simulink model "Slip_compensation_model"  (R2019b)
settings: Solver=VariableStepAuto  StartTime=0.0  StopTime=20  FixedStep=10  MaxStep=20e-3  RelTol=1e-4  EnableMultiTasking=on
undefined symbols (not defined in the file or in its folder): DiscIntNeverNeededParam, M, sigbuilder_block, slip_1, slip_2, slip_3
libraries: lib_robotinohardware x5
settings Model: EnablePacing=on  Creator=Олег  LastModifiedBy=Олег

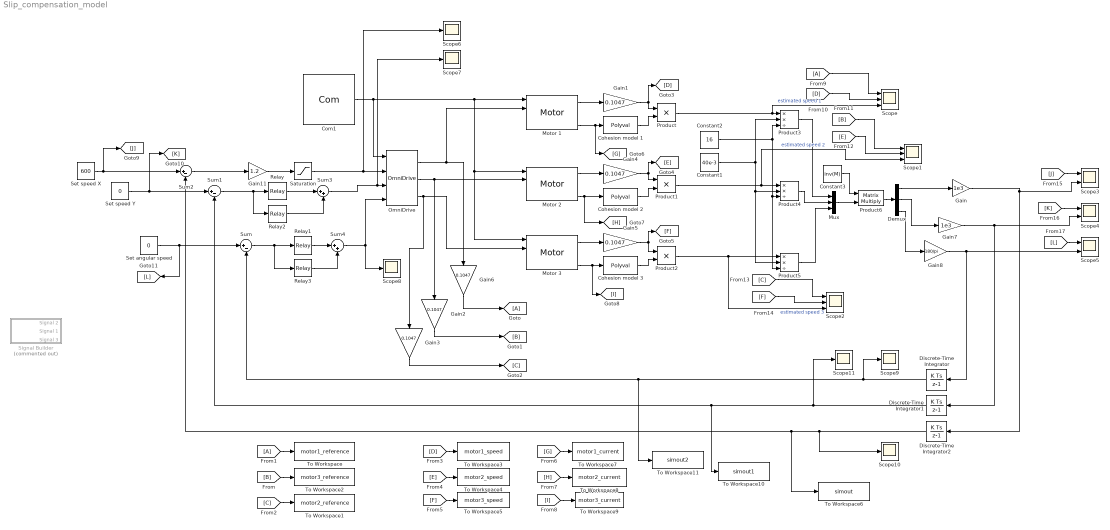
== system Slip_compensation_model ==
  Cohesion model 1 : Polyval  Coefs=slip_1
  Cohesion model 2 : Polyval  Coefs=slip_2
  Cohesion model 3 : Polyval  Coefs=slip_3
  Com1 : lib_robotinohardware/Com  ip='172.26.1.0'
  Constant1 : Constant  Value=40e-3
  Constant2 : Constant  Value=16
  Constant3 : Constant  Value=inv(M)
  Demux : Demux  Outputs=3
  Discrete-Time Integrator : DiscreteIntegrator  SampleTime=-1  ICPrevOutput=DiscIntNeverNeededParam  ICPrevScaledInput=DiscIntNeverNeededParam
  Discrete-Time Integrator1 : DiscreteIntegrator  SampleTime=-1  ICPrevOutput=DiscIntNeverNeededParam  ICPrevScaledInput=DiscIntNeverNeededParam
  Discrete-Time Integrator2 : DiscreteIntegrator  SampleTime=-1  ICPrevOutput=DiscIntNeverNeededParam  ICPrevScaledInput=DiscIntNeverNeededParam
  Gain : Gain  Gain=1e3
  Gain{1..6} (6 alike) : Gain  Gain=0.1047
  Gain11 : Gain  Gain=1.2
  Gain7 : Gain  Gain=1e3
  Gain8 : Gain  Gain=180/pi
  Motor 1 : lib_robotinohardware/Motor  num=0  kp=200  ki=10  kd=0
  Motor 2 : lib_robotinohardware/Motor  num=1  kp=200  ki=10  kd=0
  Motor 3 : lib_robotinohardware/Motor  num=2  kp=200  ki=10  kd=0
  Mux : Mux  Inputs=3
  OmniDrive : lib_robotinohardware/OmniDrive
  Product : Product
  Product1 : Product
  Product2 : Product
  Product3 : Product  Inputs=**/
  Product4 : Product  Inputs=**/
  Product5 : Product  Inputs=**/
  Product6 : Product  Multiplication=Matrix(*)
  Relay : Relay  OnSwitchValue=3  OffSwitchValue=1.5  OnOutputValue=30
  Relay1 : Relay  OnSwitchValue=1  OffSwitchValue=0.5  OnOutputValue=20
  Relay2 : Relay  OnSwitchValue=-1.5  OffSwitchValue=-3  OnOutputValue=0  OffOutputValue=-30
  Relay3 : Relay  OnSwitchValue=-0.5  OffSwitchValue=-1  OnOutputValue=0  OffOutputValue=-20
  Saturation : Saturate  UpperLimit=300  LowerLimit=-300
  Scope : Scope  NumInputPorts=3
  Scope1 : Scope  NumInputPorts=3
  Scope{6..11} (6 alike) : Scope
  Scope2 : Scope  NumInputPorts=3
  Scope3 : Scope  NumInputPorts=2
  Scope4 : Scope  NumInputPorts=2
  Scope5 : Scope  NumInputPorts=2
  Set angular speed : Constant  Value=0
  Set speed X : Constant  Value=600
  Set speed Y : Constant  Value=0
  Signal Builder : Subsystem  Tag=STV Subsys  Commented=on  LoadFcn=sigbuilder_block('load');  StartFcn=sigbuilder_block('start');  StopFcn=sigbuilder_block('stop');  ClipboardFcn=sigbuilder_block('clipboard');  mask(Sigbuilder block){tuvar=[0:10]}
      mask help: Simulink:masks:SigbuilderBlock_MD
      mask init:
      | if ~strcmp(get_param(bdroot(gcbh),'SimulationStatus'),'stopped') tuvar = sigbuilder_block('maskInit'); end
      settings: CopyFcn=sigbuilder_block('copy');  DeleteFcn=sigbuilder_block('delete');  ModelCloseFcn=sigbuilder_block('modelClose');  PreSaveFcn=sigbuilder_block('preSave');  PauseFcn=sigbuilder_block('pause');  ContinueFcn=sigbuilder_block('continue');  NameChangeFcn=sigbuilder_block('namechange');  OpenFcn=sigbuilder_block('open',[5.4 30 1141.2 522.6 ]);  CloseFcn=sigbuilder_block('close');
      mask Display: plot(0, 0, 100, 100,[2, 2, 32, 32, 2], [68, 8, 8, 68, 68],[32, 2], [38, 38], [32, 19, 2],[53, 60, 44], [32, 17, 17, 2],[16, 16, 31, 31]);txt = getActiveGroup(gcbh);text(2, 100, txt,'verticalAlignment', 'top');
  Sum : Sum  Inputs=|+-
  Sum1 : Sum  Inputs=|+-
  Sum2 : Sum  Inputs=|+-
  Sum3 : Sum  Inputs=|++
  Sum4 : Sum  Inputs=|++
  To Workspace : ToWorkspace  VariableName=motor1_reference  SaveFormat=Timeseries  SampleTime=-1
  To Workspace1 : ToWorkspace  VariableName=motor2_reference  SaveFormat=Timeseries  SampleTime=-1
  To Workspace10 : ToWorkspace  VariableName=simout1  SaveFormat=Timeseries  SampleTime=-1
  To Workspace11 : ToWorkspace  VariableName=simout2  SaveFormat=Timeseries  SampleTime=-1
  To Workspace2 : ToWorkspace  VariableName=motor3_reference  SaveFormat=Timeseries  SampleTime=-1
  To Workspace3 : ToWorkspace  VariableName=motor1_speed  SaveFormat=Timeseries  SampleTime=-1
  To Workspace4 : ToWorkspace  VariableName=motor2_speed  SaveFormat=Timeseries  SampleTime=-1
  To Workspace5 : ToWorkspace  VariableName=motor3_speed  SaveFormat=Timeseries  SampleTime=-1
  To Workspace6 : ToWorkspace  VariableName=simout  SaveFormat=Timeseries  SampleTime=-1
  To Workspace7 : ToWorkspace  VariableName=motor1_current  SaveFormat=Timeseries  SampleTime=-1
  To Workspace8 : ToWorkspace  VariableName=motor2_current  SaveFormat=Timeseries  SampleTime=-1
  To Workspace9 : ToWorkspace  VariableName=motor3_current  SaveFormat=Timeseries  SampleTime=-1
  wires:
  Com1/1 -> OmniDrive/1, Motor 1/1, Motor 3/1, Motor 2/1
  OmniDrive/2 -> Gain2/1, Motor 2/2
  OmniDrive/1 -> Gain6/1, Motor 1/2
  OmniDrive/3 -> Gain3/1, Motor 3/2
  Gain3/1 -> [C]
  Gain6/1 -> [A]
  Motor 3/1 -> Gain5/1
  Motor 2/1 -> Gain4/1
  Motor 1/1 -> Gain1/1
  Gain2/1 -> [B]
  Motor 1/3 -> [G], Cohesion model 1/1
  Motor 2/3 -> [H], Cohesion model 2/1
  Motor 3/3 -> [I], Cohesion model 3/1
  Gain1/1 -> [D], Product/1
  Cohesion model 1/1 -> Product/2
  Gain4/1 -> [E], Product1/1
  Cohesion model 2/1 -> Product1/2
  Gain5/1 -> [F], Product2/1
  Cohesion model 3/1 -> Product2/2
  Set speed X/1 -> [J], Sum2/1
  Sum2/1 -> Gain11/1
  Set speed Y/1 -> [K], Sum1/1
  Set angular speed/1 -> [L], Sum/1
  Sum1/1 -> Relay2/1, Relay/1
  Constant1/1 -> Product3/2, Product5/2, Product4/2
  Product6/1 -> Demux/1
  Constant2/1 -> Product5/3, Product4/3, Product3/3
  Product3/1 -> Mux/1
  Mux/1 -> Product6/2
  Constant3/1 -> Product6/1
  Product5/1 -> Mux/3
  Product4/1 -> Mux/2
  Product/1 -> Scope/3, Product3/1  "estimated speed 1"
  Product1/1 -> Scope1/3, Product4/1  "estimated speed 2"
  Product2/1 -> Scope2/3, Product5/1  "estimated speed 3"
  Demux/3 -> Gain8/1
  Demux/2 -> Gain7/1
  Demux/1 -> Gain/1
  [A] -> To Workspace/1
  [B] -> To Workspace2/1
  [C] -> To Workspace1/1
  [D] -> To Workspace3/1
  [E] -> To Workspace4/1
  [F] -> To Workspace5/1
  [G] -> To Workspace7/1
  [H] -> To Workspace8/1
  [I] -> To Workspace9/1
  [A] -> Scope/1
  [D] -> Scope/2
  [B] -> Scope1/1
  [E] -> Scope1/2
  [C] -> Scope2/1
  [F] -> Scope2/2
  [J] -> Scope3/1
  [K] -> Scope4/1
  [L] -> Scope5/1
  Gain/1 -> Discrete-Time Integrator2/1, Scope3/2
  Gain7/1 -> Discrete-Time Integrator1/1, Scope4/2
  Gain8/1 -> Discrete-Time Integrator/1, Scope5/2
  Discrete-Time Integrator/1 -> To Workspace11/1, Sum/2, Scope9/1
  Discrete-Time Integrator1/1 -> To Workspace10/1, Sum1/2, Scope11/1
  Discrete-Time Integrator2/1 -> Scope10/1, To Workspace6/1, Sum2/2
  Gain11/1 -> Saturation/1
  Saturation/1 -> Scope6/1, OmniDrive/2
  Sum/1 -> Relay3/1, Relay1/1
  Relay/1 -> Sum3/1
  Relay2/1 -> Sum3/2
  Sum3/1 -> Scope7/1, OmniDrive/3
  Relay1/1 -> Sum4/1
  Sum4/1 -> Scope8/1, OmniDrive/4
  Relay3/1 -> Sum4/2

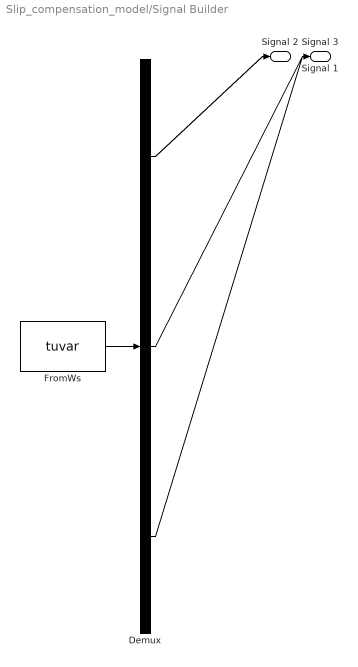
== system Slip_compensation_model/Signal Builder ==
  Demux : Demux  Tag=STV Demux  Outputs=3
  FromWs : FromWorkspace  Tag=STV FromWs  VariableName=tuvar  SampleTime=0
      SigBuilderData=|
      | common.afterFinalStr = 'Extrapolate'
      | common.sampleTime = 0
      | dataSet.timeRange = [0 180]
      | dataSet.name = 'Group 1'
      | sbobj.Groups.Name = 'Group 1'
      | sbobj.Groups.Signals(1).Name = 'Signal 2'
      | sbobj.Groups.Signals(1).XData = [0 1 1 7.4 7.4 9.6 9.6 13.6 13.6 20 20 26 26 30.8 30.8 35.8 35.8 40 40 43.8 43.8 48.2 48.2 57.4 57.4 180]
      | sbobj.Groups.Signals(1).YData = [0 0 100 100 0 0 -300 -300 0 0 200 200 0 0 -200 -200 0 0 300 300 0 0 -100 -100 0 0]
      | sbobj.Groups.Signals(2).Name = 'Signal 1'
      | sbobj.Groups.Signals(2).XData = [0 8.57142857143 59.2 59.2 66.4 66.4 70.6 70.6 74.6 74.6 81.4 81.4 88.6 88.6 93.4 93.4 99.4 99.4 103.6 103.6 107.8 107.8 111.6 111.6 119 119 180]
      | sbobj.Groups.Signals(2).YData = [0 0 0 100 100 0 0 -300 -300 0 0 200 200 0 0 -200 -200 0 0 300 300 0 0 -100 -100 0 0]
      | sbobj.Groups.Signals(3).Name = 'Signal 3'
      | sbobj.Groups.Signals(3).XData = [0 8.57142857143 123 123 131.6 131.6 134.8 134.8 140 140 143.4 143.4 148.6 148.6 153 153 159.2 159.2 163 163 168.6 168.6 171.6 171.6 179 179 180]
      | sbobj.Groups.Signals(3).YData = [0 0 0 20 20 0 0 -40 -40 0 0 30 30 0 0 -30 -30 0 0 40 40 0 0 -20 -20 0 0]
      | sbobj.Groups.TimeRange = [0 180]
  Signal 2 : Outport  Tag=STV Outport
  Signal 1 : Outport  Tag=STV Outport  Port=2
  Signal 3 : Outport  Tag=STV Outport  Port=3
  wires:
  FromWs/1 -> Demux/1
  Demux/1 -> Signal 2/1
  Demux/2 -> Signal 1/1
  Demux/3 -> Signal 3/1
